simulink model "Vending_machine_model"  (R2020b)
settings: Solver=VariableStepAuto  StartTime=0.0  StopTime=10  RelTol=1e-3
settings Model: Creator=HP  LastModifiedBy=HP

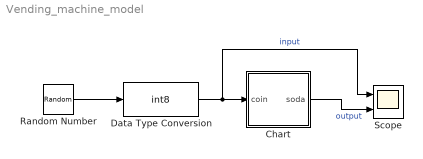
== system Vending_machine_model ==
  Chart : Stateflow chart  TreatAsAtomicUnit=on
  Data Type Conversion : DataTypeConversion  OutDataTypeStr=int8  RndMeth=Nearest
  Random Number : RandomNumber  SampleTime=0.1
  Scope : Scope  NumInputPorts=2
  wires:
  Random Number/1 -> Data Type Conversion/1
  Data Type Conversion/1 -> Scope/1, Chart/1(coin)  "input"
  Chart/1(soda) -> Scope/2  "output"

== stateflow chart Vending_machine_model/Chart ==
  state got_0
  state got_nickel
  state got_dime
  (default) -> got_0
  got_0 -> got_nickel [order 1] : [coin==1]{soda=0}
  got_nickel -> got_0 [order 1] : [coin==2]{soda=1}
  got_0 -> got_dime [order 2] : [coin==2]{soda=0}
  got_dime -> got_0 [order 1] : [coin==1]{soda=1}
  got_nickel -> got_dime [order 2] : [coin==1]{soda=0}
  got_dime -> got_nickel [order 2] : [coin==2]{soda=1}
  data: coin input; soda output
